simulink model "SimOrbit"  (R2015a)
settings: Solver=ode3  StartTime=0.0  StopTime=86400  FixedStep=120  RelTol=1e-3
values from neighbouring files (symbols this model uses):
  a = - sqrt( (L^2-2*T*Iy) / ((Ix-Iy)*Ix) )    [polhodeAnalytical.m]
  M = (3*mu)/(R^3) * [(Iz - Iy)*cy*cz ... (first row only)    [grav_grad.m]    (also in int_Euler_eqs_grav.m)
  M0 = grav_grad(vsr.I_princ,vsr.mu,r_princ)    [propagate_attitude.m]
undefined symbols (not defined in the file or in its folder): D, dUT1, e, i, n, Om, w, Y
settings Model: Creator=Kaitlin  LastModifiedBy=Kaitlin

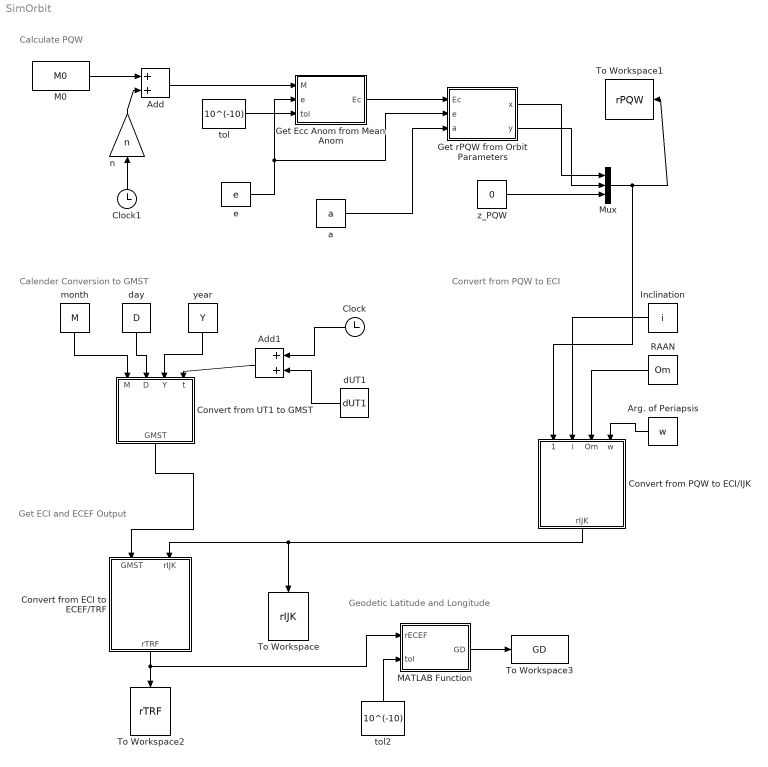
== system SimOrbit ==
  note: Geodetic Latitude and Longitude
  note: Get ECI and ECEF Output
  note: Calculate PQW
  note: Convert from PQW to ECI
  note: Calender Conversion to GMST
  Add : Sum
  Add1 : Sum
  Arg. of Periapsis : Constant  Value=w
  Clock : Clock
  Clock1 : Clock
  Convert from ECI to ECEF/TRF : MATLAB Function  TreatAsAtomicUnit=on
  Convert from PQW to ECI/IJK : MATLAB Function  TreatAsAtomicUnit=on
  Convert from UT1 to GMST : MATLAB Function  TreatAsAtomicUnit=on
  Get Ecc Anom from Mean Anom : MATLAB Function  TreatAsAtomicUnit=on
  Get rPQW from Orbit Parameters : MATLAB Function  TreatAsAtomicUnit=on
  Inclination : Constant  Value=i
  M0 : Constant  Value=M0
  MATLAB Function : MATLAB Function  TreatAsAtomicUnit=on
  Mux : Mux  Inputs=3
  RAAN : Constant  Value=Om
  To Workspace : ToWorkspace  VariableName=rIJK  SampleTime=-1
      settings: Save2DSignal=2-D array (concatenate along first dimension)
  To Workspace1 : ToWorkspace  VariableName=rPQW  SampleTime=-1
      settings: Save2DSignal=2-D array (concatenate along first dimension)
  To Workspace2 : ToWorkspace  VariableName=rTRF  SampleTime=-1
      settings: Save2DSignal=2-D array (concatenate along first dimension)
  To Workspace3 : ToWorkspace  VariableName=GD  SampleTime=-1
  a : Constant  Value=a
  dUT1 : Constant  Value=dUT1
  day : Constant  Value=D
  e : Constant  Value=e
  month : Constant  Value=M
  n : Gain  Gain=n
  tol : Constant  Value=10^(-10)
  tol2 : Constant  Value=10^(-10)
  year : Constant  Value=Y
  z_PQW : Constant  Value=0
  wires:
  M0/1 -> Add/1
  n/1 -> Add/2
  Add/1 -> Get Ecc Anom from Mean Anom/1(M)
  tol/1 -> Get Ecc Anom from Mean Anom/3(tol)
  Get Ecc Anom from Mean Anom/1(Ec) -> Get rPQW from Orbit Parameters/1(Ec)
  Get rPQW from Orbit Parameters/1(x) -> Mux/1
  Get rPQW from Orbit Parameters/2(y) -> Mux/2
  z_PQW/1 -> Mux/3
  Convert from UT1 to GMST/1(GMST) -> Convert from ECI to ECEF/TRF/1(GMST)
  Convert from ECI to ECEF/TRF/1(rTRF) -> MATLAB Function/1(rECEF), To Workspace2/1
  a/1 -> Get rPQW from Orbit Parameters/3(a)
  e/1 -> Get rPQW from Orbit Parameters/2(e), Get Ecc Anom from Mean Anom/2(e)
  Convert from PQW to ECI/IJK/1(rIJK) -> To Workspace/1, Convert from ECI to ECEF/TRF/2(rIJK)
  Inclination/1 -> Convert from PQW to ECI/IJK/2(i)
  Mux/1 -> Convert from PQW to ECI/IJK/1(rPQW), To Workspace1/1
  month/1 -> Convert from UT1 to GMST/1(M)
  day/1 -> Convert from UT1 to GMST/2(D)
  year/1 -> Convert from UT1 to GMST/3(Y)
  tol2/1 -> MATLAB Function/2(tol)
  MATLAB Function/1(GD) -> To Workspace3/1
  Clock1/1 -> n/1
  Add1/1 -> Convert from UT1 to GMST/4(t)
  dUT1/1 -> Add1/2
  Clock/1 -> Add1/1
  Arg. of Periapsis/1 -> Convert from PQW to ECI/IJK/4(w)
  RAAN/1 -> Convert from PQW to ECI/IJK/3(Om)

== matlab function SimOrbit/Get rPQW from Orbit Parameters ==
  data: x output; Ec input; y output; e input; a input
function [x,y] = EctoPos(Ec,e,a)
x = a*(cos(Ec)-e);
y = a*sqrt(1-e^2)*sin(Ec);
end

== matlab function SimOrbit/Get Ecc Anom from Mean Anom ==
  data: M input; Ec output; e input; tol input
function Ec = fcn(M,e,tol)
er = 100;
Ec = M;
Eco = M;
iter = 0;
while er >= tol && iter <= 100
    del = -(Eco-e*sin(Eco)-M)/(1-e*cos(Eco));
    Ec = Eco + del;
    er = abs(Ec-Eco);
    Eco = Ec;
    iter = iter + 1;
end

== matlab function SimOrbit/Convert from PQW to ECI//IJK ==
  data: rPQW input; rIJK output; i input; Om input; w input
function rIJK  = rIJKsim(rPQW,i,Om,w)
R = rotPQWtoIJK(Om,i,w);
rIJK = R*rPQW;
end

== matlab function SimOrbit/Convert from UT1 to GMST ==
  data: M input; GMST output; D input; Y input; t input
function GMST = GMSTsim(M,D,Y,t)
MJD = UT1toMJD(M,D,Y,t);
GMST = MJDtoGMST(MJD);
end

== matlab function SimOrbit/Convert from ECI to ECEF//TRF ==
  data: GMST input; rTRF output; rIJK input
function rTRF  = rTRFsim(GMST,rIJK)
R = rotCRFtoTRF(GMST);
rTRF = R*rIJK;
end

== matlab function SimOrbit/MATLAB Function ==
  data: rECEF input; GD output; tol input
function GD = fcn(rECEF,tol)
imax = 100;
GD = ECEFtoGD(rECEF,tol,imax)';
end
